simulink model "zcoilControlDesign"  (R2024a)
settings: Solver=VariableStepAuto  StartTime=0.0  StopTime=1000  RelTol=1e-3
undefined symbols (not defined in the file or in its folder): ref, x, z
settings Model: Creator=workstation  LastModifiedBy=workstation
settings DataIOCC: SaveFormat=Array

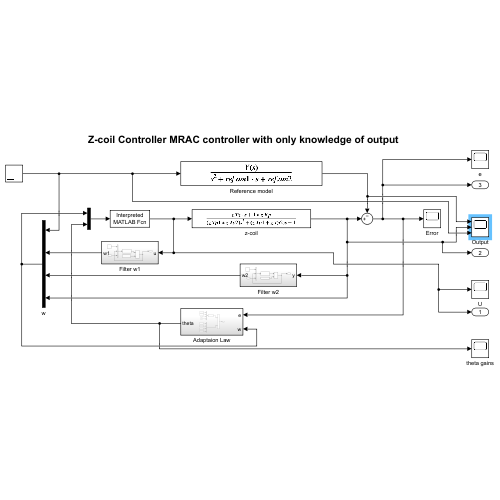
[thumbnail: Simulink's stored preview of the top-level diagram]
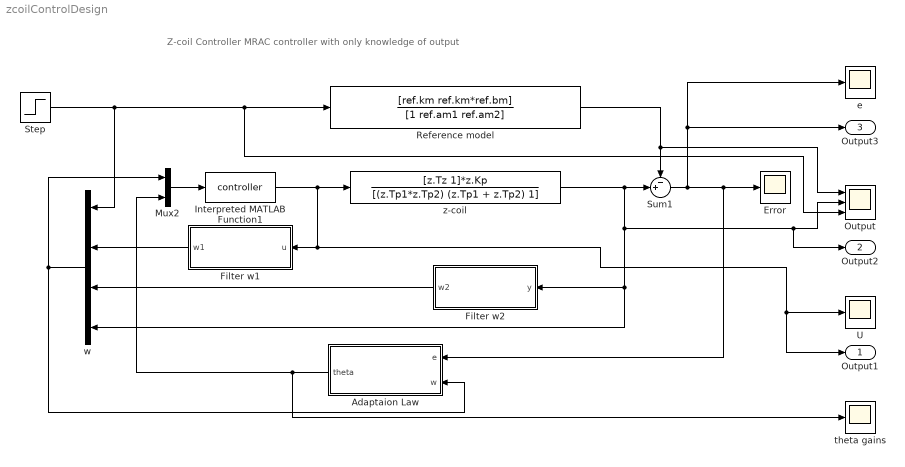
== system zcoilControlDesign ==
  note: Z-coil Controller MRAC controller with only knowledge of output
  Adaptaion Law : Subsystem
  Error : Scope
  Filter w1 : Subsystem
  Filter w2 : Subsystem
  Interpreted MATLAB Function1 : MATLABFcn  MATLABFcn=controller  OutputDimensions=1
  Mux2 : Mux  Inputs=2
  Output : Scope  NumInputPorts=3
  Reference model : TransferFcn  Numerator=[ref.km ref.km*ref.bm]  Denominator=[1 ref.am1 ref.am2]
  Step : Step  Time=1E-3  SampleTime=0
  Sum1 : Sum  Inputs=-+|
  U : Scope
  e : Scope
  theta gains : Scope
  w : Mux
  z-coil : TransferFcn  Numerator=[z.Tz 1]*z.Kp  Denominator=[(z.Tp1*z.Tp2) (z.Tp1 + z.Tp2) 1]
  Output1 : Outport
  Output2 : Outport  Port=2
  Output3 : Outport  Port=3
  wires:
  Adaptaion Law/1(theta) -> theta gains/1, Mux2/2
  z-coil/1 -> w/4, Filter w2/1(y), Output2/1, Output/2, Sum1/2
  Reference model/1 -> Output/1, Sum1/1
  Mux2/1 -> Interpreted MATLAB Function1/1
  Step/1 -> w/1, Output/3, Reference model/1
  Sum1/1 -> e/1, Output3/1, Adaptaion Law/1(e), Error/1
  Filter w1/1(w1) -> w/2
  Filter w2/1(w2) -> w/3
  w/1 -> Mux2/1, Adaptaion Law/2(w)
  Interpreted MATLAB Function1/1 -> Output1/1, U/1, Filter w1/1(u), z-coil/1

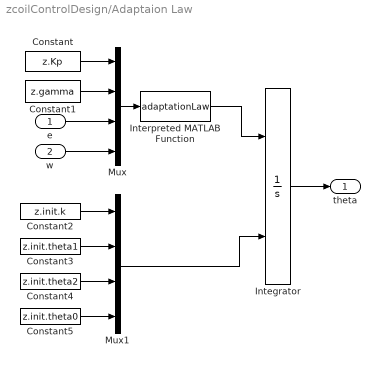
== system zcoilControlDesign/Adaptaion Law ==
  e : Inport
  w : Inport  Port=2
  Constant : Constant  Value=z.Kp
  Constant1 : Constant  Value=z.gamma
  Constant2 : Constant  Value=z.init.k
  Constant3 : Constant  Value=z.init.theta1
  Constant4 : Constant  Value=z.init.theta2
  Constant5 : Constant  Value=z.init.theta0
  Integrator : Integrator  InitialConditionSource=external  InitialCondition=[ref.km/x.Kp,2e-6,2e-6,2e-6]
  Interpreted MATLAB Function : MATLABFcn  MATLABFcn=adaptationLaw  OutputDimensions=4
  Mux : Mux
  Mux1 : Mux
  theta : Outport
  wires:
  Constant1/1 -> Mux/2
  e/1 -> Mux/3
  w/1 -> Mux/4
  Constant/1 -> Mux/1
  Mux/1 -> Interpreted MATLAB Function/1
  Interpreted MATLAB Function/1 -> Integrator/1
  Integrator/1 -> theta/1
  Mux1/1 -> Integrator/2
  Constant2/1 -> Mux1/1
  Constant3/1 -> Mux1/2
  Constant4/1 -> Mux1/3
  Constant5/1 -> Mux1/4

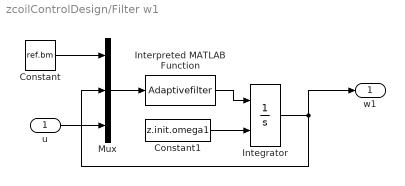
== system zcoilControlDesign/Filter w1 ==
  u : Inport
  Constant : Constant  Value=ref.bm
  Constant1 : Constant  Value=z.init.omega1
  Integrator : Integrator  InitialConditionSource=external  InitialCondition=0.1
  Interpreted MATLAB Function : MATLABFcn  MATLABFcn=Adaptivefilter  OutputDimensions=1
  Mux : Mux  Inputs=3
  w1 : Outport
  wires:
  u/1 -> Mux/3
  Constant/1 -> Mux/1
  Interpreted MATLAB Function/1 -> Integrator/1
  Mux/1 -> Interpreted MATLAB Function/1
  Integrator/1 -> w1/1, Mux/2
  Constant1/1 -> Integrator/2

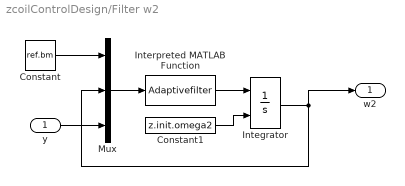
== system zcoilControlDesign/Filter w2 ==
  y : Inport
  Constant : Constant  Value=ref.bm
  Constant1 : Constant  Value=z.init.omega2
  Integrator : Integrator  InitialConditionSource=external  InitialCondition=0.1
  Interpreted MATLAB Function : MATLABFcn  MATLABFcn=Adaptivefilter  OutputDimensions=1
  Mux : Mux  Inputs=3
  w2 : Outport
  wires:
  y/1 -> Mux/3
  Constant/1 -> Mux/1
  Interpreted MATLAB Function/1 -> Integrator/1
  Mux/1 -> Interpreted MATLAB Function/1
  Integrator/1 -> w2/1, Mux/2
  Constant1/1 -> Integrator/2
